simulink model "homework2_5"  (R2016a)
settings: Solver=ode1  StartTime=0.0  StopTime=0.056  FixedStep=0.001  RelTol=1e-3
model workspace (MAT data in the model file):
  C = 0.001
  R = 1000
  U = 5
settings Model: Creator=chris.barlow  LastModifiedBy=chris.barlow

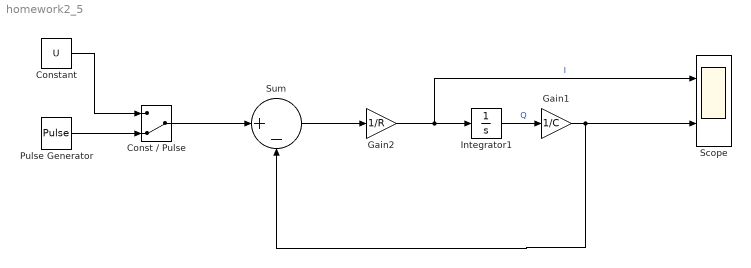
== system homework2_5 ==
  Const / Pulse : ManualSwitch  CurrentSetting=0
  Constant : Constant  Value=U
  Gain1 : Gain  Gain=1/C
  Gain2 : Gain  Gain=1/R
  Integrator1 : Integrator
  Pulse Generator : DiscretePulseGenerator  PulseType=Time based  Amplitude=U  Period=10  PulseWidth=50
  Scope : Scope  NumInputPorts=2
  Sum : Sum  Inputs=|+-
  wires:
  Const / Pulse/1 -> Sum/1
  Gain2/1 -> Scope/1, Integrator1/1  "I"
  Sum/1 -> Gain2/1
  Integrator1/1 -> Gain1/1  "Q"
  Gain1/1 -> Scope/2, Sum/2
  Pulse Generator/1 -> Const / Pulse/2
  Constant/1 -> Const / Pulse/1
